simulink model "project"  (R2024b)
settings: Solver=VariableStepAuto  StartTime=0.0  StopTime=(size(Xp,2)-1)*dt  MaxStep=0.01  RelTol=1e-3
values from neighbouring files (symbols this model uses):
  Ic = I    (= 0)    [quadcopter_tmp_par.m]
  m = 4    [inertia.m]    (also in quadcopter_tmp_par.m)
  M_RB = [ m*eye(3) , zeros(3) ; zeros(3) , Ic2 ]    [inertia.m]    (also in quadcopter_tmp_par.m = [m*eye(3),zeros(3);zeros(3),Ic])
undefined symbols (not defined in the file or in its folder): alpha_P, alpha_X, alpha_Y, alpha_Z
libraries: sharedtransform x2, simulink_extras x1, sharedutil x1
settings Model: Creator=fildo7525  LastModifiedBy=vince

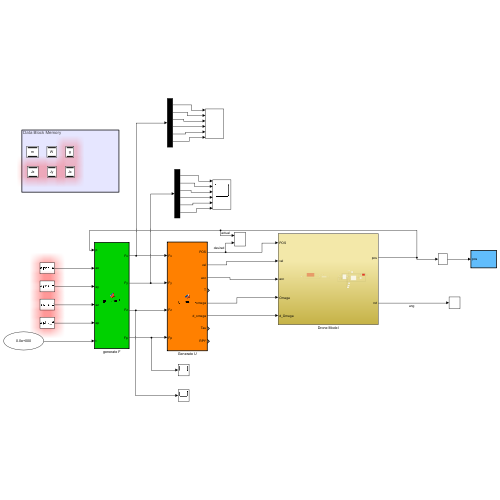
[thumbnail: Simulink's stored preview of the top-level diagram]
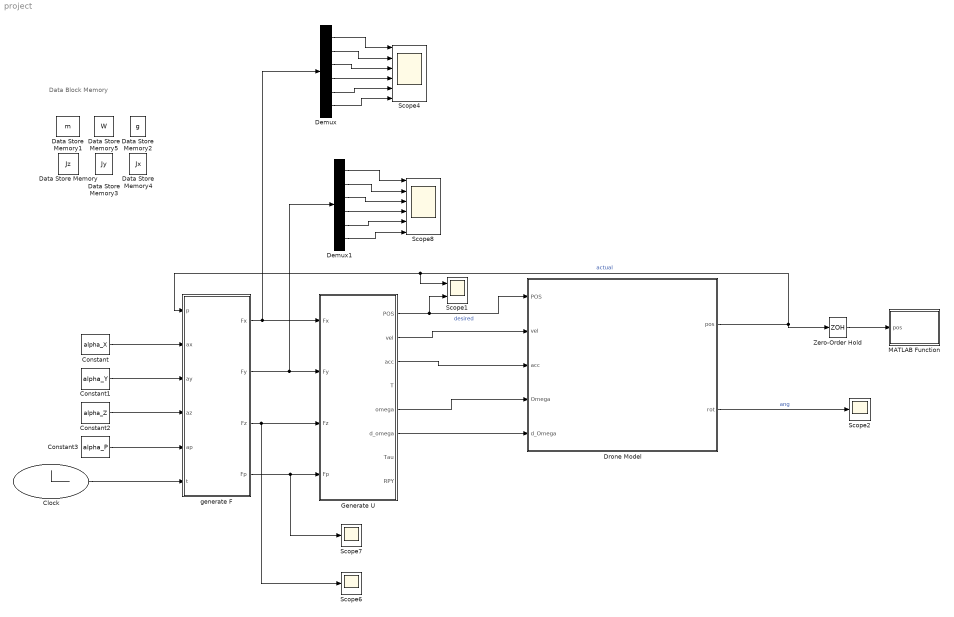
== system project ==
  note: Data Block Memory
  Clock : Clock
  Constant : Constant  Value=alpha_X
  Constant1 : Constant  Value=alpha_Y
  Constant2 : Constant  Value=alpha_Z
  Constant3 : Constant  Value=alpha_P
  Data Store Memory : DataStoreMemory  DataStoreName=Jz  WriteAfterWriteMsg=warning  InitialValue=Jz  ShowAdditionalParam=off  OutDataTypeStr=double
  Data Store Memory1 : DataStoreMemory  DataStoreName=m  WriteAfterWriteMsg=warning  InitialValue=m  ShowAdditionalParam=off  OutDataTypeStr=double
  Data Store Memory2 : DataStoreMemory  DataStoreName=g  WriteAfterWriteMsg=warning  InitialValue=g  ShowAdditionalParam=off  OutDataTypeStr=double
  Data Store Memory3 : DataStoreMemory  DataStoreName=Jy  WriteAfterWriteMsg=warning  InitialValue=Jy  ShowAdditionalParam=off  OutDataTypeStr=double
  Data Store Memory4 : DataStoreMemory  DataStoreName=Jx  WriteAfterWriteMsg=warning  InitialValue=Jx  ShowAdditionalParam=off  OutDataTypeStr=double
  Data Store Memory5 : DataStoreMemory  DataStoreName=W  WriteAfterWriteMsg=warning  InitialValue=W  ShowAdditionalParam=off  OutDataTypeStr=double
  Demux : Demux  Outputs=6
  Demux1 : Demux  Outputs=6
  Drone Model : Subsystem
  Generate U : MATLAB Function  TreatAsAtomicUnit=on
  MATLAB Function : MATLAB Function  TreatAsAtomicUnit=on
  Scope1 : Scope  NumInputPorts=2
  Scope2 : Scope
  Scope4 : Scope  NumInputPorts=6
  Scope6 : Scope
  Scope7 : Scope
  Scope8 : Scope  NumInputPorts=6
  Zero-Order Hold : ZeroOrderHold  SampleTime=0.1
  generate F : MATLAB Function  TreatAsAtomicUnit=on
  wires:
  Constant2/1 -> generate F/4(az)
  generate F/2(Fy) -> Demux1/1, Generate U/2(Fy)
  generate F/1(Fx) -> Demux/1, Generate U/1(Fx)
  Clock/1 -> generate F/6(t)
  Constant3/1 -> generate F/5(ap)
  generate F/3(Fz) -> Scope6/1, Generate U/3(Fz)
  Constant1/1 -> generate F/3(ay)
  generate F/4(Fp) -> Scope7/1, Generate U/4(Fp)
  Constant/1 -> generate F/2(ax)
  Demux/6 -> Scope4/6
  Demux/1 -> Scope4/1
  Demux/2 -> Scope4/2
  Demux/3 -> Scope4/3
  Demux/4 -> Scope4/4
  Demux/5 -> Scope4/5
  Demux1/4 -> Scope8/4
  Demux1/3 -> Scope8/3
  Demux1/1 -> Scope8/1
  Demux1/2 -> Scope8/2
  Demux1/5 -> Scope8/5
  Demux1/6 -> Scope8/6
  Drone Model/1(pos) -> Zero-Order Hold/1, Scope1/1, generate F/1(p)  "actual"
  Zero-Order Hold/1 -> MATLAB Function/1(pos)
  Drone Model/2(rot) -> Scope2/1  "ang"
  Generate U/1(POS) -> Scope1/2, Drone Model/1(POS)  "desired"
  Generate U/5(omega) -> Drone Model/4(Omega)
  Generate U/2(vel) -> Drone Model/2(vel)
  Generate U/3(acc) -> Drone Model/3(acc)
  Generate U/6(d_omega) -> Drone Model/5(d_Omega)

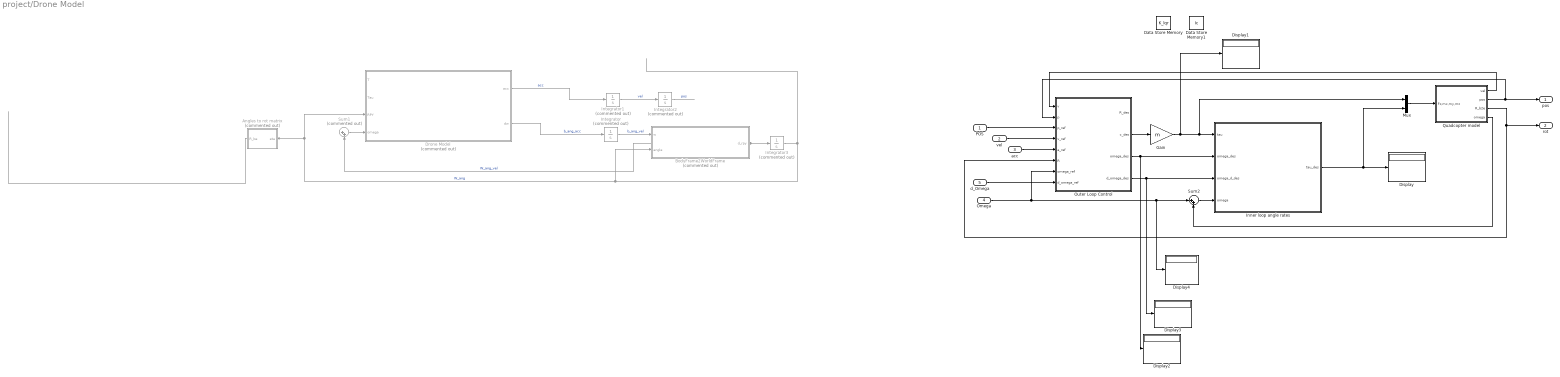
== system project/Drone Model ==
  POS : Inport
  vel : Inport  Port=2
  acc : Inport  Port=3
  Omega : Inport  Port=4
  d_Omega : Inport  Port=5
  Angles to rot matrix : MATLAB Function  Commented=on  TreatAsAtomicUnit=on
  BodyFrame2WorldFrame : MATLAB Function  Commented=on  TreatAsAtomicUnit=on
  Data Store Memory : DataStoreMemory  DataStoreName=K_lqr  WriteAfterWriteMsg=warning  InitialValue=K_lqr  VectorParams1D=off  ShowAdditionalParam=off  OutDataTypeStr=double
  Data Store Memory1 : DataStoreMemory  DataStoreName=Ic  WriteAfterWriteMsg=warning  InitialValue=Ic  VectorParams1D=off  ShowAdditionalParam=off  OutDataTypeStr=double
  Display{,1..4} (5 alike) : Display
  Drone Model : MATLAB Function  Commented=on  TreatAsAtomicUnit=on
  Gain : Gain  Gain=m
  Inner loop angle rates : MATLAB Function  TreatAsAtomicUnit=on
  Integrator{,1..3} (4 alike) : Integrator  Commented=on  InitialCondition=zeros(3,1)
  Mux : Mux  Inputs=2
  Outer Loop Control : MATLAB Function  TreatAsAtomicUnit=on
  Quadcopter model : Subsystem
  Sum1 : Sum  Commented=on  Inputs=|++
  Sum2 : Sum  Inputs=|++
  pos : Outport
  rot : Outport  Port=2
  wires:
  Integrator2/1 -> ?  "pos"
  Drone Model/1(acc) -> Integrator1/1  "acc"
  Drone Model/2(dw) -> Integrator/1  "b_ang_acc"
  Integrator1/1 -> Integrator2/1  "vel"
  BodyFrame2WorldFrame/1(d_rpy) -> Integrator3/1, Sum1/2  "W_ang_vel"
  Integrator3/1 -> Drone Model/3(RPY), Angles to rot matrix/1(eta), BodyFrame2WorldFrame/2(angle)  "W_ang"
  Integrator/1 -> BodyFrame2WorldFrame/1(w)  "b_ang_vel"
  Sum1/1 -> Drone Model/4(omega)
  Omega/1 -> Display4/1, Sum2/1, Outer Loop Control/7(omega_ref)
  POS/1 -> Outer Loop Control/3(p_ref)
  vel/1 -> Outer Loop Control/4(v_ref)
  acc/1 -> Outer Loop Control/5(a_ref)
  Angles to rot matrix/1(R_be) -> ?
  Outer Loop Control/3(omega_des) -> Inner loop angle rates/2(omega_des), Display2/1
  Outer Loop Control/4(d_omega_des) -> Display3/1, Inner loop angle rates/3(omega_d_des)
  Inner loop angle rates/1(tau_des) -> Mux/2, Display/1
  Outer Loop Control/2(c_des) -> Gain/1
  Gain/1 -> Display1/1, Mux/1, Inner loop angle rates/1(tau)
  Mux/1 -> Quadcopter model/1(Fz,mx,my,mz)
  Quadcopter model/2(pos) -> pos/1, Outer Loop Control/2(p)
  Quadcopter model/1(vel) -> Outer Loop Control/1(v)
  Quadcopter model/3(R_b2e) -> rot/1, Outer Loop Control/6(R)
  Quadcopter model/4(omega) -> Sum2/2
  Sum2/1 -> Inner loop angle rates/4(omega)
  d_Omega/1 -> Outer Loop Control/8(d_omega_ref)

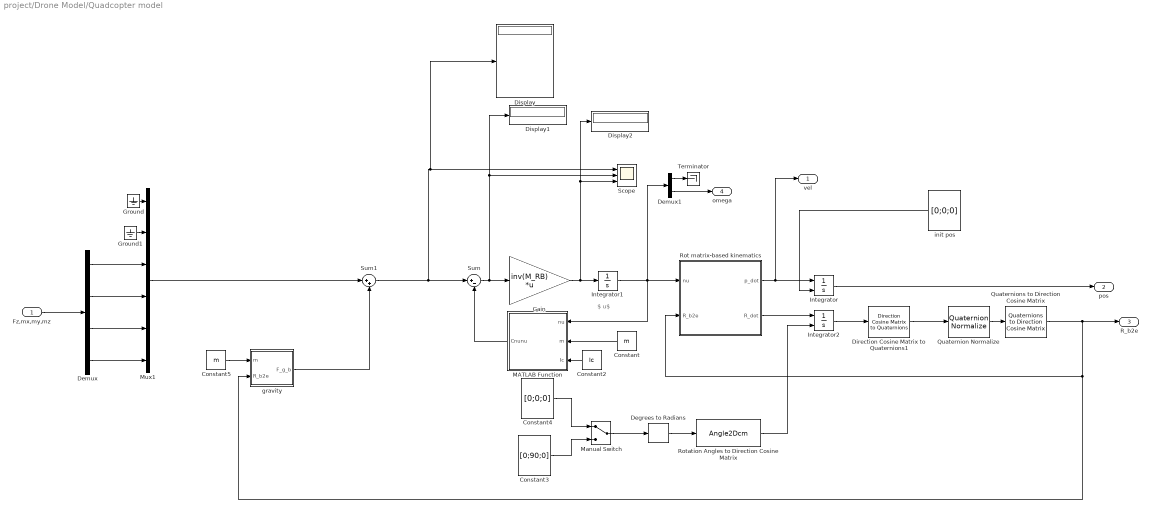
== system project/Drone Model/Quadcopter model ==
  note: $\nu$
  Fz,mx,my,mz : Inport
  Constant : Constant  Value=m
  Constant2 : Constant  Value=Ic  VectorParams1D=off
  Constant3 : Constant  Value=[0;90;0]  VectorParams1D=off
  Constant4 : Constant  Value=[0;0;0]  VectorParams1D=off
  Constant5 : Constant  Value=m
  Degrees to Radians : simulink_extras/Transformations/Degrees to Radians
  Demux : Demux
  Demux1 : Demux  Outputs=2
  Direction Cosine Matrix to Quaternions1 : sharedtransform/Direction Cosine Matrix  to Quaternions  aMode=0  action=None  tolerance=eps(2)
  Display : Display
      settings: Decimation=3
  Display1 : Display
      settings: Decimation=3
  Display2 : Display
      settings: Decimation=3
  Gain : Gain  Gain=inv(M_RB)  Multiplication=Matrix(K*u) (u vector)
  Ground : Ground
  Ground1 : Ground
  Integrator : Integrator  InitialConditionSource=external  InitialCondition=[0;0;-10]
  Integrator1 : Integrator  InitialCondition=[0;0;0;0;0;0]
  Integrator2 : Integrator  InitialConditionSource=external  InitialCondition=[0;0;-10;0;pi/2;0]
  MATLAB Function : MATLAB Function  TreatAsAtomicUnit=on
  Manual Switch : ManualSwitch
  Mux1 : Mux  Inputs=6
  Quaternion Normalize : sharedutil/Quaternion Normalize  aMode=aMode
  Quaternions to Direction Cosine Matrix : sharedtransform/Quaternions to  Direction Cosine Matrix  aMode=aMode
  Rot matrix-based kinematics : Subsystem
  Rotation Angles to Direction Cosine Matrix : Angle2Dcm
      settings: AttributesFormatString=Rotation Order: %<rotationOrder>
  Scope : Scope  NumInputPorts=3
  Sum : Sum  Inputs=|+-
  Sum1 : Sum  Inputs=|++
  Terminator : Terminator
  gravity : MATLAB Function  TreatAsAtomicUnit=on
  init pos : Constant  Value=[0;0;0]  VectorParams1D=off
  vel : Outport
  pos : Outport  Port=2
  R_b2e : Outport  Port=3
  omega : Outport  Port=4
  wires:
  Constant/1 -> MATLAB Function/2(m)
  Degrees to Radians/1 -> Rotation Angles to Direction Cosine Matrix/1
  Constant2/1 -> MATLAB Function/3(Ic)
  init pos/1 -> Integrator/2
  Constant4/1 -> Manual Switch/1
  MATLAB Function/1(Cnunu) -> Sum/2
  Gain/1 -> Display2/1, Scope/3, Integrator1/1
  Constant3/1 -> Manual Switch/2
  Rotation Angles to Direction Cosine Matrix/1 -> Integrator2/2
  Sum/1 -> Scope/2, Display1/1, Gain/1
  Manual Switch/1 -> Degrees to Radians/1
  Rot matrix-based kinematics/1(p_dot) -> Integrator/1, vel/1
  Rot matrix-based kinematics/2(R_dot) -> Integrator2/1
  Integrator/1 -> pos/1
  Demux/4 -> Mux1/6
  Demux/3 -> Mux1/5
  Demux/2 -> Mux1/4
  Fz,mx,my,mz/1 -> Demux/1
  Ground/1 -> Mux1/1
  Ground1/1 -> Mux1/2
  Quaternion Normalize/1 -> Quaternions to Direction Cosine Matrix/1
  Constant5/1 -> gravity/1(m)
  gravity/1(F_g_b) -> Sum1/2
  Sum1/1 -> Display/1, Scope/1, Sum/1
  Demux/1 -> Mux1/3
  Integrator1/1 -> Demux1/1, MATLAB Function/1(nu), Rot matrix-based kinematics/1(nu)
  Direction Cosine Matrix to Quaternions1/1 -> Quaternion Normalize/1
  Quaternions to Direction Cosine Matrix/1 -> gravity/2(R_b2e), Rot matrix-based kinematics/2(R_b2e), R_b2e/1
  Integrator2/1 -> Direction Cosine Matrix to Quaternions1/1
  Mux1/1 -> Sum1/1
  Demux1/1 -> Terminator/1
  Demux1/2 -> omega/1

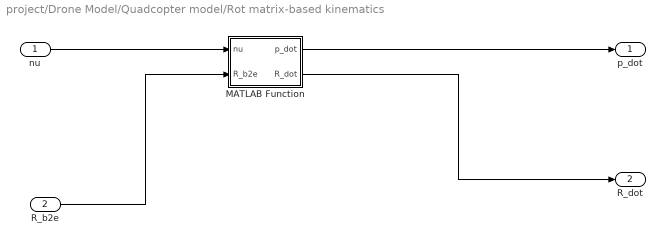
== system project/Drone Model/Quadcopter model/Rot matrix-based kinematics ==
  nu : Inport
  R_b2e : Inport  Port=2
  MATLAB Function : MATLAB Function  TreatAsAtomicUnit=on
  p_dot : Outport
  R_dot : Outport  Port=2
  wires:
  MATLAB Function/2(R_dot) -> R_dot/1
  nu/1 -> MATLAB Function/1(nu)
  R_b2e/1 -> MATLAB Function/2(R_b2e)
  MATLAB Function/1(p_dot) -> p_dot/1

== matlab function project/Drone Model/Angles to rot matrix ==
  data: R_be output; eta input
function R_be = fcn(eta)

% Euler angle extraction
phi = eta(4);
theta = eta(5);
psi = eta(6);

R_xphi = [ 1 0 0 ; 0 cos(phi) -sin(phi) ; 0 sin(phi) cos(phi) ];
R_ytheta = [ cos(theta) 0 sin(theta) ; 0 1 0 ; -sin(theta) 0 cos(theta) ];
R_zpsi = [ cos(psi) -sin(psi) 0 ; sin(psi) cos(psi) 0 ; 0 0 1 ];

% rotation matrix
R_be = R_zpsi * R_ytheta * R_xphi;

== matlab function project/Drone Model/BodyFrame2WorldFrame ==
  data: d_rpy output; w input; angle input
function d_rpy = convertBodyFrame2WorldFrame(w, angle)
	Fi = angle(1);
	Theta = angle(2);
	Psi = angle(3);

	R = [1, 0		, -sin(Theta);
		 0, cos(Fi) , cos(Theta)*sin(Fi);
		 0, -sin(Fi), cos(Theta)*cos(Fi)];

	d_rpy = R \ w;

== matlab function project/Drone Model/Quadcopter model/MATLAB Function ==
  data: nu input; Cnunu output; m input; Ic input
function Cnunu = fcn(nu,m,Ic)

v = nu(1:3);  % linear velocities (expressed in the body frame)
omega = nu(4:6); % angular velocities (expressed in the body frame)

% Coriolis term
Cnunu = [ cross(omega,m*v) ; -cross(Ic*omega,omega) ];

== matlab function project/Drone Model/Quadcopter model/gravity ==
  data: m input; R_b2e input; F_g_b output
function F_g_b = fcn(m,R_b2e)
F_g=[0;0;-m*9.81];
F_g_b=[R_b2e'*F_g;0;0;0];

== matlab function project/Drone Model/Quadcopter model/Rot matrix-based kinematics/MATLAB Function ==
  data: nu input; p_dot output; R_b2e input; R_dot output
function [p_dot,R_dot] = fcn(nu,R_b2e)
v_b=nu(1:3);
w_b=nu(4:6);
p_dot=R_b2e*v_b;
omega_cross=[0,-w_b(3),w_b(2);
             w_b(3),0,-w_b(1);
             -w_b(2),w_b(1),0];
R_dot=R_b2e*omega_cross;

== matlab function project/Drone Model/Inner loop angle rates ==
  settings: updateMethod=DISCRETE
  data: tau input; omega_des input; omega_d_des input; omega input; tau_des output; Ic data_store_memory; K_lqr data_store_memory
function tau_des = inner(tau, omega_des, omega_d_des, omega)
	global K_lqr;
	global Ic;

	tau_ref = cross(omega_des, Ic*omega_des) + Ic*omega_d_des;
	
	tau_des = K_lqr * [omega_des-omega; tau_ref-tau] + cross(omega, Ic*omega) + Ic * omega_d_des;

== matlab function project/generate F ==
  settings: updateMethod=DISCRETE
  data: p input; ax input; Fx output; ay input; az input; ap input; t input; Fy output; Fz output; Fp output; W data_store_memory
function [Fx, Fy, Fz, Fp] = generateF(p, ax, ay, az, ap, t)
    global W;
    
    persistent acceptance;
	persistent idx;

    if isempty(idx)
		idx = 1;
        % acceptance = 0.2;
		acceptance = 0.5;
    end

	b0 = [ 1 ; t ; t^2	; t^3	; t^4	 ; t^5];
	b1 = [ 0 ; 1 ; 2*t	; 3*t^2 ; 4*t^3	 ; 5*t^4];
    b2 = [ 0 ; 0 ; 2	; 6*t	; 12*t^2 ; 20*t^3];
	b3 = [ 0 ; 0 ; 0	; 6		; 24*t	 ; 60*t^2];
	b4 = [ 0 ; 0 ; 0	; 0		; 24	 ; 120*t];
	b5 = [ 0 ; 0 ; 0	; 0		; 0		 ; 120];
    
    Fx = [ax(idx, :)*b0; ax(idx, :)*b1; ax(idx, :)*b2; ax(idx, :)*b3; ax(idx, :)*b4; ax(idx, :)*b5];
    Fy = [ay(idx, :)*b0; ay(idx, :)*b1; ay(idx, :)*b2; ay(idx, :)*b3; ay(idx, :)*b4; ay(idx, :)*b5];
    Fz = [az(idx, :)*b0; az(idx, :)*b1; az(idx, :)*b2; az(idx, :)*b3; az(idx, :)*b4; az(idx, :)*b5];
    Fp = [ap(idx, :)*b0; ap(idx, :)*b1; ap(idx, :)*b2; ap(idx, :)*b3; ap(idx, :)*b4; ap(idx, :)*b5];

    %v = K*(pd - p) Fi,
	dif = norm(W(idx+1, 1:3) - p');
    if dif <= acceptance
		if idx + 1 < size(W, 1)
			idx = idx + 1;
		end
	end

end

== matlab function project/Generate U ==
  data: POS output; vel output; acc output; Fx input; T output; omega output; d_omega output; Tau output; RPY output; Fy input; Fz input; Fp input; Jz data_store_memory; g data_store_memory; m data_store_memory; Jx data_store_memory; Jy data_store_memory
function [POS, vel, acc, T, omega, d_omega, Tau, RPY] = generateU(Fx, Fy, Fz, Fp)
    global Jz;
    global Jy;
    global Jx;
    global m;
    global g;
    
    f1c4f2s4 = Fx(3) * cos(Fp(1)) + Fy(3) * sin(Fp(1));
    
    T = m * sqrt( Fx(3)^2 + Fy(3)^2 + (Fz(3) + g)^2 );
	POS = [Fx(1); Fy(1); Fz(1)];
	vel = [Fx(1); Fy(1); Fz(1)];
	acc = [Fx(1); Fy(1); Fz(1)];
	
	Psi = Fp(1);
	tmp = Fx(3)*cos(Psi) + Fy(3)*sin(Psi);
	Theta = atan2( tmp, Fz(3) + g );
	Fi = atan2( Fx(3)*sin(Psi) - Fy(3)*cos(Psi), sqrt( (Fz(3)+g)^2 + tmp^2) );
	
	RPY = [ Fi; Theta; Psi];


	wx = ((sin(Fp(1))*Fx(4) - cos(Fp(1))*Fy(4) + cos(Fp(1))*Fx(3)*Fp(2) + sin(Fp(1))*Fy(3)*Fp(2))/((Fz(3) + g)^2 + (cos(Fp(1))*Fx(3) + sin(Fp(1))*Fy(3))^2)^(1/2) + ((2*(Fz(3) + g)*Fz(4) + 2*(cos(Fp(1))*Fx(3) + sin(Fp(1))*Fy(3))*(sin(Fp(1))*Fy(4) + cos(Fp(1))*Fx(4) + cos(Fp(1))*Fy(3)*Fp(2) - sin(Fp(1))*Fx(3)*Fp(2)))*(cos(Fp(1))*Fy(3) - sin(Fp(1))*Fx(3)))/(2*((Fz(3) + g)^2 + (cos(Fp(1))*Fx(3) + sin(Fp(1))*Fy(3))^2)^(3/2)))/((cos(Fp(1))*Fy(3) - sin(Fp(1))*Fx(3))^2/((Fz(3) + g)^2 + (cos(Fp(1))*Fx(3) + sin(Fp(1))*Fy(3))^2) + 1) - ((cos(Fp(1))*Fx(3) + sin(Fp(1))*Fy(3))*Fp(2))/(((cos(Fp(1))*Fx(3) + sin(Fp(1))*Fy(3))^2/(Fz(3) + g)^2 + 1)^(1/2)*(Fz(3) + g));
	wy = ((sin(Fp(1))*Fy(4) + cos(Fp(1))*Fx(4) + cos(Fp(1))*Fy(3)*Fp(2) - sin(Fp(1))*Fx(3)*Fp(2))/(Fz(3) + g) - ((cos(Fp(1))*Fx(3) + sin(Fp(1))*Fy(3))*Fz(4))/(Fz(3) + g)^2)/(((cos(Fp(1))*Fx(3) + sin(Fp(1))*Fy(3))^2/(Fz(3) + g)^2 + 1)*((cos(Fp(1))*Fy(3) - sin(Fp(1))*Fx(3))^2/((Fz(3) + g)^2 + (cos(Fp(1))*Fx(3) + sin(Fp(1))*Fy(3))^2) + 1)^(1/2)) - ((cos(Fp(1))*Fy(3) - sin(Fp(1))*Fx(3))*Fp(2))/(((cos(Fp(1))*Fx(3) + sin(Fp(1))*Fy(3))^2/(Fz(3) + g)^2 + 1)^(1/2)*((cos(Fp(1))*Fy(3) - sin(Fp(1))*Fx(3))^2/((Fz(3) + g)^2 + (cos(Fp(1))*Fx(3) + sin(Fp(1))*Fy(3))^2) + 1)^(1/2)*((Fz(3) + g)^2 + (cos(Fp(1))*Fx(3) + sin(Fp(1))*Fy(3))^2)^(1/2));
	wz = Fp(2)/(((cos(Fp(1))*Fx(3) + sin(Fp(1))*Fy(3))^2/(Fz(3) + g)^2 + 1)^(1/2)*((cos(Fp(1))*Fy(3) - sin(Fp(1))*Fx(3))^2/((Fz(3) + g)^2 + (cos(Fp(1))*Fx(3) + sin(Fp(1))*Fy(3))^2) + 1)^(1/2)) + (((sin(Fp(1))*Fy(4) + cos(Fp(1))*Fx(4) + cos(Fp(1))*Fy(3)*Fp(2) - sin(Fp(1))*Fx(3)*Fp(2))/(Fz(3) + g) - ((cos(Fp(1))*Fx(3) + sin(Fp(1))*Fy(3))*Fz(4))/(Fz(3) + g)^2)*(cos(Fp(1))*Fy(3) - sin(Fp(1))*Fx(3)))/(((cos(Fp(1))*Fx(3) + sin(Fp(1))*Fy(3))^2/(Fz(3) + g)^2 + 1)*((cos(Fp(1))*Fy(3) - sin(Fp(1))*Fx(3))^2/((Fz(3) + g)^2 + (cos(Fp(1))*Fx(3) + sin(Fp(1))*Fy(3))^2) + 1)^(1/2)*((Fz(3) + g)^2 + (cos(Fp(1))*Fx(3) + sin(Fp(1))*Fy(3))^2)^(1/2));

	omega = [wx; wy; wz];

	dwx = ((sin(Fp(1))*Fx(5) - cos(Fp(1))*Fy(5) + cos(Fp(1))*Fp(2)^2*Fy(3) - sin(Fp(1))*Fp(2)^2*Fx(3) + 2*cos(Fp(1))*Fp(2)*Fx(4) + cos(Fp(1))*Fp(3)*Fx(3) + 2*sin(Fp(1))*Fp(2)*Fy(4) + sin(Fp(1))*Fp(3)*Fy(3))/((Fz(3) + g)^2 + (cos(Fp(1))*Fx(3) + sin(Fp(1))*Fy(3))^2)^(1/2) + ((cos(Fp(1))*Fy(3) - sin(Fp(1))*Fx(3))*(2*(cos(Fp(1))*Fx(3) + sin(Fp(1))*Fy(3))*(cos(Fp(1))*Fx(5) + sin(Fp(1))*Fy(5) - cos(Fp(1))*Fp(2)^2*Fx(3) - sin(Fp(1))*Fp(2)^2*Fy(3) + 2*cos(Fp(1))*Fp(2)*Fy(4) + cos(Fp(1))*Fp(3)*Fy(3) - 2*sin(Fp(1))*Fp(2)*Fx(4) - sin(Fp(1))*Fp(3)*Fx(3)) + 2*(Fz(3) + g)*Fz(5) + 2*Fz(4)^2 + 2*(sin(Fp(1))*Fy(4) + cos(Fp(1))*Fx(4) + cos(Fp(1))*Fy(3)*Fp(2) - sin(Fp(1))*Fx(3)*Fp(2))^2))/(2*((Fz(3) + g)^2 + (cos(Fp(1))*Fx(3) + sin(Fp(1))*Fy(3))^2)^(3/2)) - ((2*(Fz(3) + g)*Fz(4) + 2*(cos(Fp(1))*Fx(3) + sin(Fp(1))*Fy(3))*(sin(Fp(1))*Fy(4) + cos(Fp(1))*Fx(4) + cos(Fp(1))*Fy(3)*Fp(2) - sin(Fp(1))*Fx(3)*Fp(2)))*(sin(Fp(1))*Fx(4) - cos(Fp(1))*Fy(4) + cos(Fp(1))*Fx(3)*Fp(2) + sin(Fp(1))*Fy(3)*Fp(2)))/((Fz(3) + g)^2 + (cos(Fp(1))*Fx(3) + sin(Fp(1))*Fy(3))^2)^(3/2) - (3*(2*(Fz(3) + g)*Fz(4) + 2*(cos(Fp(1))*Fx(3) + sin(Fp(1))*Fy(3))*(sin(Fp(1))*Fy(4) + cos(Fp(1))*Fx(4) + cos(Fp(1))*Fy(3)*Fp(2) - sin(Fp(1))*Fx(3)*Fp(2)))^2*(cos(Fp(1))*Fy(3) - sin(Fp(1))*Fx(3)))/(4*((Fz(3) + g)^2 + (cos(Fp(1))*Fx(3) + sin(Fp(1))*Fy(3))^2)^(5/2)))/((cos(Fp(1))*Fy(3) - sin(Fp(1))*Fx(3))^2/((Fz(3) + g)^2 + (cos(Fp(1))*Fx(3) + sin(Fp(1))*Fy(3))^2) + 1) + (((sin(Fp(1))*Fx(4) - cos(Fp(1))*Fy(4) + cos(Fp(1))*Fx(3)*Fp(2) + sin(Fp(1))*Fy(3)*Fp(2))/((Fz(3) + g)^2 + (cos(Fp(1))*Fx(3) + sin(Fp(1))*Fy(3))^2)^(1/2) + ((2*(Fz(3) + g)*Fz(4) + 2*(cos(Fp(1))*Fx(3) + sin(Fp(1))*Fy(3))*(sin(Fp(1))*Fy(4) + cos(Fp(1))*Fx(4) + cos(Fp(1))*Fy(3)*Fp(2) - sin(Fp(1))*Fx(3)*Fp(2)))*(cos(Fp(1))*Fy(3) - sin(Fp(1))*Fx(3)))/(2*((Fz(3) + g)^2 + (cos(Fp(1))*Fx(3) + sin(Fp(1))*Fy(3))^2)^(3/2)))*(((2*(Fz(3) + g)*Fz(4) + 2*(cos(Fp(1))*Fx(3) + sin(Fp(1))*Fy(3))*(sin(Fp(1))*Fy(4) + cos(Fp(1))*Fx(4) + cos(Fp(1))*Fy(3)*Fp(2) - sin(Fp(1))*Fx(3)*Fp(2)))*(cos(Fp(1))*Fy(3) - sin(Fp(1))*Fx(3))^2)/((Fz(3) + g)^2 + (cos(Fp(1))*Fx(3) + sin(Fp(1))*Fy(3))^2)^2 + (2*(cos(Fp(1))*Fy(3) - sin(Fp(1))*Fx(3))*(sin(Fp(1))*Fx(4) - cos(Fp(1))*Fy(4) + cos(Fp(1))*Fx(3)*Fp(2) + sin(Fp(1))*Fy(3)*Fp(2)))/((Fz(3) + g)^2 + (cos(Fp(1))*Fx(3) + sin(Fp(1))*Fy(3))^2)))/((cos(Fp(1))*Fy(3) - sin(Fp(1))*Fx(3))^2/((Fz(3) + g)^2 + (cos(Fp(1))*Fx(3) + sin(Fp(1))*Fy(3))^2) + 1)^2 - (Fp(2)*(sin(Fp(1))*Fy(4) + cos(Fp(1))*Fx(4) + cos(Fp(1))*Fy(3)*Fp(2) - sin(Fp(1))*Fx(3)*Fp(2)))/(((cos(Fp(1))*Fx(3) + sin(Fp(1))*Fy(3))^2/(Fz(3) + g)^2 + 1)^(1/2)*(Fz(3) + g)) - ((cos(Fp(1))*Fx(3) + sin(Fp(1))*Fy(3))*Fp(3))/(((cos(Fp(1))*Fx(3) + sin(Fp(1))*Fy(3))^2/(Fz(3) + g)^2 + 1)^(1/2)*(Fz(3) + g)) + ((cos(Fp(1))*Fx(3) + sin(Fp(1))*Fy(3))*Fp(2)*Fz(4))/(((cos(Fp(1))*Fx(3) + sin(Fp(1))*Fy(3))^2/(Fz(3) + g)^2 + 1)^(1/2)*(Fz(3) + g)^2) + (((2*(cos(Fp(1))*Fx(3) + sin(Fp(1))*Fy(3))*(sin(Fp(1))*Fy(4) + cos(Fp(1))*Fx(4) + cos(Fp(1))*Fy(3)*Fp(2) - sin(Fp(1))*Fx(3)*Fp(2)))/(Fz(3) + g)^2 - (2*(cos(Fp(1))*Fx(3) + sin(Fp(1))*Fy(3))^2*Fz(4))/(Fz(3) + g)^3)*(cos(Fp(1))*Fx(3) + sin(Fp(1))*Fy(3))*Fp(2))/(2*((cos(Fp(1))*Fx(3) + sin(Fp(1))*Fy(3))^2/(Fz(3) + g)^2 + 1)^(3/2)*(Fz(3) + g));
	dwy = ((cos(Fp(1))*Fx(5) + sin(Fp(1))*Fy(5) - cos(Fp(1))*Fp(2)^2*Fx(3) - sin(Fp(1))*Fp(2)^2*Fy(3) + 2*cos(Fp(1))*Fp(2)*Fy(4) + cos(Fp(1))*Fp(3)*Fy(3) - 2*sin(Fp(1))*Fp(2)*Fx(4) - sin(Fp(1))*Fp(3)*Fx(3))/(Fz(3) + g) - (2*Fz(4)*(sin(Fp(1))*Fy(4) + cos(Fp(1))*Fx(4) + cos(Fp(1))*Fy(3)*Fp(2) - sin(Fp(1))*Fx(3)*Fp(2)))/(Fz(3) + g)^2 + (2*(cos(Fp(1))*Fx(3) + sin(Fp(1))*Fy(3))*Fz(4)^2)/(Fz(3) + g)^3 - ((cos(Fp(1))*Fx(3) + sin(Fp(1))*Fy(3))*Fz(5))/(Fz(3) + g)^2)/(((cos(Fp(1))*Fx(3) + sin(Fp(1))*Fy(3))^2/(Fz(3) + g)^2 + 1)*((cos(Fp(1))*Fy(3) - sin(Fp(1))*Fx(3))^2/((Fz(3) + g)^2 + (cos(Fp(1))*Fx(3) + sin(Fp(1))*Fy(3))^2) + 1)^(1/2)) + (((sin(Fp(1))*Fy(4) + cos(Fp(1))*Fx(4) + cos(Fp(1))*Fy(3)*Fp(2) - sin(Fp(1))*Fx(3)*Fp(2))/(Fz(3) + g) - ((cos(Fp(1))*Fx(3) + sin(Fp(1))*Fy(3))*Fz(4))/(Fz(3) + g)^2)*(((2*(Fz(3) + g)*Fz(4) + 2*(cos(Fp(1))*Fx(3) + sin(Fp(1))*Fy(3))*(sin(Fp(1))*Fy(4) + cos(Fp(1))*Fx(4) + cos(Fp(1))*Fy(3)*Fp(2) - sin(Fp(1))*Fx(3)*Fp(2)))*(cos(Fp(1))*Fy(3) - sin(Fp(1))*Fx(3))^2)/((Fz(3) + g)^2 + (cos(Fp(1))*Fx(3) + sin(Fp(1))*Fy(3))^2)^2 + (2*(cos(Fp(1))*Fy(3) - sin(Fp(1))*Fx(3))*(sin(Fp(1))*Fx(4) - cos(Fp(1))*Fy(4) + cos(Fp(1))*Fx(3)*Fp(2) + sin(Fp(1))*Fy(3)*Fp(2)))/((Fz(3) + g)^2 + (cos(Fp(1))*Fx(3) + sin(Fp(1))*Fy(3))^2)))/(2*((cos(Fp(1))*Fx(3) + sin(Fp(1))*Fy(3))^2/(Fz(3) + g)^2 + 1)*((cos(Fp(1))*Fy(3) - sin(Fp(1))*Fx(3))^2/((Fz(3) + g)^2 + (cos(Fp(1))*Fx(3) + sin(Fp(1))*Fy(3))^2) + 1)^(3/2)) - (((2*(cos(Fp(1))*Fx(3) + sin(Fp(1))*Fy(3))*(sin(Fp(1))*Fy(4) + cos(Fp(1))*Fx(4) + cos(Fp(1))*Fy(3)*Fp(2) - sin(Fp(1))*Fx(3)*Fp(2)))/(Fz(3) + g)^2 - (2*(cos(Fp(1))*Fx(3) + sin(Fp(1))*Fy(3))^2*Fz(4))/(Fz(3) + g)^3)*((sin(Fp(1))*Fy(4) + cos(Fp(1))*Fx(4) + cos(Fp(1))*Fy(3)*Fp(2) - sin(Fp(1))*Fx(3)*Fp(2))/(Fz(3) + g) - ((cos(Fp(1))*Fx(3) + sin(Fp(1))*Fy(3))*Fz(4))/(Fz(3) + g)^2))/(((cos(Fp(1))*Fx(3) + sin(Fp(1))*Fy(3))^2/(Fz(3) + g)^2 + 1)^2*((cos(Fp(1))*Fy(3) - sin(Fp(1))*Fx(3))^2/((Fz(3) + g)^2 + (cos(Fp(1))*Fx(3) + sin(Fp(1))*Fy(3))^2) + 1)^(1/2)) - ((cos(Fp(1))*Fy(3) - sin(Fp(1))*Fx(3))*Fp(3))/(((cos(Fp(1))*Fx(3) + sin(Fp(1))*Fy(3))^2/(Fz(3) + g)^2 + 1)^(1/2)*((cos(Fp(1))*Fy(3) - sin(Fp(1))*Fx(3))^2/((Fz(3) + g)^2 + (cos(Fp(1))*Fx(3) + sin(Fp(1))*Fy(3))^2) + 1)^(1/2)*((Fz(3) + g)^2 + (cos(Fp(1))*Fx(3) + sin(Fp(1))*Fy(3))^2)^(1/2)) + (Fp(2)*(sin(Fp(1))*Fx(4) - cos(Fp(1))*Fy(4) + cos(Fp(1))*Fx(3)*Fp(2) + sin(Fp(1))*Fy(3)*Fp(2)))/(((cos(Fp(1))*Fx(3) + sin(Fp(1))*Fy(3))^2/(Fz(3) + g)^2 + 1)^(1/2)*((cos(Fp(1))*Fy(3) - sin(Fp(1))*Fx(3))^2/((Fz(3) + g)^2 + (cos(Fp(1))*Fx(3) + sin(Fp(1))*Fy(3))^2) + 1)^(1/2)*((Fz(3) + g)^2 + (cos(Fp(1))*Fx(3) + sin(Fp(1))*Fy(3))^2)^(1/2)) - ((cos(Fp(1))*Fy(3) - sin(Fp(1))*Fx(3))*Fp(2)*(((2*(Fz(3) + g)*Fz(4) + 2*(cos(Fp(1))*Fx(3) + sin(Fp(1))*Fy(3))*(sin(Fp(1))*Fy(4) + cos(Fp(1))*Fx(4) + cos(Fp(1))*Fy(3)*Fp(2) - sin(Fp(1))*Fx(3)*Fp(2)))*(cos(Fp(1))*Fy(3) - sin(Fp(1))*Fx(3))^2)/((Fz(3) + g)^2 + (cos(Fp(1))*Fx(3) + sin(Fp(1))*Fy(3))^2)^2 + (2*(cos(Fp(1))*Fy(3) - sin(Fp(1))*Fx(3))*(sin(Fp(1))*Fx(4) - cos(Fp(1))*Fy(4) + cos(Fp(1))*Fx(3)*Fp(2) + sin(Fp(1))*Fy(3)*Fp(2)))/((Fz(3) + g)^2 + (cos(Fp(1))*Fx(3) + sin(Fp(1))*Fy(3))^2)))/(2*((cos(Fp(1))*Fx(3) + sin(Fp(1))*Fy(3))^2/(Fz(3) + g)^2 + 1)^(1/2)*((cos(Fp(1))*Fy(3) - sin(Fp(1))*Fx(3))^2/((Fz(3) + g)^2 + (cos(Fp(1))*Fx(3) + sin(Fp(1))*Fy(3))^2) + 1)^(3/2)*((Fz(3) + g)^2 + (cos(Fp(1))*Fx(3) + sin(Fp(1))*Fy(3))^2)^(1/2)) + (((2*(cos(Fp(1))*Fx(3) + sin(Fp(1))*Fy(3))*(sin(Fp(1))*Fy(4) + cos(Fp(1))*Fx(4) + cos(Fp(1))*Fy(3)*Fp(2) - sin(Fp(1))*Fx(3)*Fp(2)))/(Fz(3) + g)^2 - (2*(cos(Fp(1))*Fx(3) + sin(Fp(1))*Fy(3))^2*Fz(4))/(Fz(3) + g)^3)*(cos(Fp(1))*Fy(3) - sin(Fp(1))*Fx(3))*Fp(2))/(2*((cos(Fp(1))*Fx(3) + sin(Fp(1))*Fy(3))^2/(Fz(3) + g)^2 + 1)^(3/2)*((cos(Fp(1))*Fy(3) - sin(Fp(1))*Fx(3))^2/((Fz(3) + g)^2 + (cos(Fp(1))*Fx(3) + sin(Fp(1))*Fy(3))^2) + 1)^(1/2)*((Fz(3) + g)^2 + (cos(Fp(1))*Fx(3) + sin(Fp(1))*Fy(3))^2)^(1/2)) + ((2*(Fz(3) + g)*Fz(4) + 2*(cos(Fp(1))*Fx(3) + sin(Fp(1))*Fy(3))*(sin(Fp(1))*Fy(4) + cos(Fp(1))*Fx(4) + cos(Fp(1))*Fy(3)*Fp(2) - sin(Fp(1))*Fx(3)*Fp(2)))*(cos(Fp(1))*Fy(3) - sin(Fp(1))*Fx(3))*Fp(2))/(2*((cos(Fp(1))*Fx(3) + sin(Fp(1))*Fy(3))^2/(Fz(3) + g)^2 + 1)^(1/2)*((cos(Fp(1))*Fy(3) - sin(Fp(1))*Fx(3))^2/((Fz(3) + g)^2 + (cos(Fp(1))*Fx(3) + sin(Fp(1))*Fy(3))^2) + 1)^(1/2)*((Fz(3) + g)^2 + (cos(Fp(1))*Fx(3) + sin(Fp(1))*Fy(3))^2)^(3/2));
	dwz = Fp(3)/(((cos(Fp(1))*Fx(3) + sin(Fp(1))*Fy(3))^2/(Fz(3) + g)^2 + 1)^(1/2)*((cos(Fp(1))*Fy(3) - sin(Fp(1))*Fx(3))^2/((Fz(3) + g)^2 + (cos(Fp(1))*Fx(3) + sin(Fp(1))*Fy(3))^2) + 1)^(1/2)) - (((2*(cos(Fp(1))*Fx(3) + sin(Fp(1))*Fy(3))*(sin(Fp(1))*Fy(4) + cos(Fp(1))*Fx(4) + cos(Fp(1))*Fy(3)*Fp(2) - sin(Fp(1))*Fx(3)*Fp(2)))/(Fz(3) + g)^2 - (2*(cos(Fp(1))*Fx(3) + sin(Fp(1))*Fy(3))^2*Fz(4))/(Fz(3) + g)^3)*Fp(2))/(2*((cos(Fp(1))*Fx(3) + sin(Fp(1))*Fy(3))^2/(Fz(3) + g)^2 + 1)^(3/2)*((cos(Fp(1))*Fy(3) - sin(Fp(1))*Fx(3))^2/((Fz(3) + g)^2 + (cos(Fp(1))*Fx(3) + sin(Fp(1))*Fy(3))^2) + 1)^(1/2)) + (Fp(2)*(((2*(Fz(3) + g)*Fz(4) + 2*(cos(Fp(1))*Fx(3) + sin(Fp(1))*Fy(3))*(sin(Fp(1))*Fy(4) + cos(Fp(1))*Fx(4) + cos(Fp(1))*Fy(3)*Fp(2) - sin(Fp(1))*Fx(3)*Fp(2)))*(cos(Fp(1))*Fy(3) - sin(Fp(1))*Fx(3))^2)/((Fz(3) + g)^2 + (cos(Fp(1))*Fx(3) + sin(Fp(1))*Fy(3))^2)^2 + (2*(cos(Fp(1))*Fy(3) - sin(Fp(1))*Fx(3))*(sin(Fp(1))*Fx(4) - cos(Fp(1))*Fy(4) + cos(Fp(1))*Fx(3)*Fp(2) + sin(Fp(1))*Fy(3)*Fp(2)))/((Fz(3) + g)^2 + (cos(Fp(1))*Fx(3) + sin(Fp(1))*Fy(3))^2)))/(2*((cos(Fp(1))*Fx(3) + sin(Fp(1))*Fy(3))^2/(Fz(3) + g)^2 + 1)^(1/2)*((cos(Fp(1))*Fy(3) - sin(Fp(1))*Fx(3))^2/((Fz(3) + g)^2 + (cos(Fp(1))*Fx(3) + sin(Fp(1))*Fy(3))^2) + 1)^(3/2)) + ((cos(Fp(1))*Fy(3) - sin(Fp(1))*Fx(3))*((cos(Fp(1))*Fx(5) + sin(Fp(1))*Fy(5) - cos(Fp(1))*Fp(2)^2*Fx(3) - sin(Fp(1))*Fp(2)^2*Fy(3) + 2*cos(Fp(1))*Fp(2)*Fy(4) + cos(Fp(1))*Fp(3)*Fy(3) - 2*sin(Fp(1))*Fp(2)*Fx(4) - sin(Fp(1))*Fp(3)*Fx(3))/(Fz(3) + g) - (2*Fz(4)*(sin(Fp(1))*Fy(4) + cos(Fp(1))*Fx(4) + cos(Fp(1))*Fy(3)*Fp(2) - sin(Fp(1))*Fx(3)*Fp(2)))/(Fz(3) + g)^2 + (2*(cos(Fp(1))*Fx(3) + sin(Fp(1))*Fy(3))*Fz(4)^2)/(Fz(3) + g)^3 - ((cos(Fp(1))*Fx(3) + sin(Fp(1))*Fy(3))*Fz(5))/(Fz(3) + g)^2))/(((cos(Fp(1))*Fx(3) + sin(Fp(1))*Fy(3))^2/(Fz(3) + g)^2 + 1)*((cos(Fp(1))*Fy(3) - sin(Fp(1))*Fx(3))^2/((Fz(3) + g)^2 + (cos(Fp(1))*Fx(3) + sin(Fp(1))*Fy(3))^2) + 1)^(1/2)*((Fz(3) + g)^2 + (cos(Fp(1))*Fx(3) + sin(Fp(1))*Fy(3))^2)^(1/2)) - (((sin(Fp(1))*Fy(4) + cos(Fp(1))*Fx(4) + cos(Fp(1))*Fy(3)*Fp(2) - sin(Fp(1))*Fx(3)*Fp(2))/(Fz(3) + g) - ((cos(Fp(1))*Fx(3) + sin(Fp(1))*Fy(3))*Fz(4))/(Fz(3) + g)^2)*(sin(Fp(1))*Fx(4) - cos(Fp(1))*Fy(4) + cos(Fp(1))*Fx(3)*Fp(2) + sin(Fp(1))*Fy(3)*Fp(2)))/(((cos(Fp(1))*Fx(3) + sin(Fp(1))*Fy(3))^2/(Fz(3) + g)^2 + 1)*((cos(Fp(1))*Fy(3) - sin(Fp(1))*Fx(3))^2/((Fz(3) + g)^2 + (cos(Fp(1))*Fx(3) + sin(Fp(1))*Fy(3))^2) + 1)^(1/2)*((Fz(3) + g)^2 + (cos(Fp(1))*Fx(3) + sin(Fp(1))*Fy(3))^2)^(1/2)) + (((sin(Fp(1))*Fy(4) + cos(Fp(1))*Fx(4) + cos(Fp(1))*Fy(3)*Fp(2) - sin(Fp(1))*Fx(3)*Fp(2))/(Fz(3) + g) - ((cos(Fp(1))*Fx(3) + sin(Fp(1))*Fy(3))*Fz(4))/(Fz(3) + g)^2)*(cos(Fp(1))*Fy(3) - sin(Fp(1))*Fx(3))*(((2*(Fz(3) + g)*Fz(4) + 2*(cos(Fp(1))*Fx(3) + sin(Fp(1))*Fy(3))*(sin(Fp(1))*Fy(4) + cos(Fp(1))*Fx(4) + cos(Fp(1))*Fy(3)*Fp(2) - sin(Fp(1))*Fx(3)*Fp(2)))*(cos(Fp(1))*Fy(3) - sin(Fp(1))*Fx(3))^2)/((Fz(3) + g)^2 + (cos(Fp(1))*Fx(3) + sin(Fp(1))*Fy(3))^2)^2 + (2*(cos(Fp(1))*Fy(3) - sin(Fp(1))*Fx(3))*(sin(Fp(1))*Fx(4) - cos(Fp(1))*Fy(4) + cos(Fp(1))*Fx(3)*Fp(2) + sin(Fp(1))*Fy(3)*Fp(2)))/((Fz(3) + g)^2 + (cos(Fp(1))*Fx(3) + sin(Fp(1))*Fy(3))^2)))/(2*((cos(Fp(1))*Fx(3) + sin(Fp(1))*Fy(3))^2/(Fz(3) + g)^2 + 1)*((cos(Fp(1))*Fy(3) - sin(Fp(1))*Fx(3))^2/((Fz(3) + g)^2 + (cos(Fp(1))*Fx(3) + sin(Fp(1))*Fy(3))^2) + 1)^(3/2)*((Fz(3) + g)^2 + (cos(Fp(1))*Fx(3) + sin(Fp(1))*Fy(3))^2)^(1/2)) - (((2*(cos(Fp(1))*Fx(3) + sin(Fp(1))*Fy(3))*(sin(Fp(1))*Fy(4) + cos(Fp(1))*Fx(4) + cos(Fp(1))*Fy(3)*Fp(2) - sin(Fp(1))*Fx(3)*Fp(2)))/(Fz(3) + g)^2 - (2*(cos(Fp(1))*Fx(3) + sin(Fp(1))*Fy(3))^2*Fz(4))/(Fz(3) + g)^3)*((sin(Fp(1))*Fy(4) + cos(Fp(1))*Fx(4) + cos(Fp(1))*Fy(3)*Fp(2) - sin(Fp(1))*Fx(3)*Fp(2))/(Fz(3) + g) - ((cos(Fp(1))*Fx(3) + sin(Fp(1))*Fy(3))*Fz(4))/(Fz(3) + g)^2)*(cos(Fp(1))*Fy(3) - sin(Fp(1))*Fx(3)))/(((cos(Fp(1))*Fx(3) + sin(Fp(1))*Fy(3))^2/(Fz(3) + g)^2 + 1)^2*((cos(Fp(1))*Fy(3) - sin(Fp(1))*Fx(3))^2/((Fz(3) + g)^2 + (cos(Fp(1))*Fx(3) + sin(Fp(1))*Fy(3))^2) + 1)^(1/2)*((Fz(3) + g)^2 + (cos(Fp(1))*Fx(3) + sin(Fp(1))*Fy(3))^2)^(1/2)) - ((2*(Fz(3) + g)*Fz(4) + 2*(cos(Fp(1))*Fx(3) + sin(Fp(1))*Fy(3))*(sin(Fp(1))*Fy(4) + cos(Fp(1))*Fx(4) + cos(Fp(1))*Fy(3)*Fp(2) - sin(Fp(1))*Fx(3)*Fp(2)))*((sin(Fp(1))*Fy(4) + cos(Fp(1))*Fx(4) + cos(Fp(1))*Fy(3)*Fp(2) - sin(Fp(1))*Fx(3)*Fp(2))/(Fz(3) + g) - ((cos(Fp(1))*Fx(3) + sin(Fp(1))*Fy(3))*Fz(4))/(Fz(3) + g)^2)*(cos(Fp(1))*Fy(3) - sin(Fp(1))*Fx(3)))/(2*((cos(Fp(1))*Fx(3) + sin(Fp(1))*Fy(3))^2/(Fz(3) + g)^2 + 1)*((cos(Fp(1))*Fy(3) - sin(Fp(1))*Fx(3))^2/((Fz(3) + g)^2 + (cos(Fp(1))*Fx(3) + sin(Fp(1))*Fy(3))^2) + 1)^(1/2)*((Fz(3) + g)^2 + (cos(Fp(1))*Fx(3) + sin(Fp(1))*Fy(3))^2)^(3/2));

	d_omega = [dwx; dwy; dwz];

    TauX = Jx*dwx + (Jz - Jy)*wy*wz;
    TauY = Jy*dwy + (Jx - Jz)*wx*wz;
    TauZ = Jz*dwz + (Jy - Jx)*wx*wy;

	Tau = [TauX; TauY; TauZ];

== matlab function project/Drone Model/Drone Model ==
  settings: updateMethod=DISCRETE
  data: T input; Tau input; RPY input; acc output; dw output; omega input; m data_store_memory; Jz data_store_memory; Jy data_store_memory; Jx data_store_memory; g data_store_memory
function [acc, dw] = drone(T, Tau, RPY, omega)
    global m;
    global g;
    global Jz;
    global Jy;
    global Jx;

	Fi = RPY(1);
	Theta = RPY(2);
	Psi = RPY(3);

	TauX = Tau(1);
	TauY = Tau(2);
	TauZ = Tau(3);

	wx = omega(1);
	wy = omega(2);
	wz = omega(3);

	x_dd = T / m * ( cos(Psi)*sin(Theta)*cos(Fi) + sin(Psi)*sin(Fi) );
	y_dd = T / m * ( sin(Psi)*sin(Theta)*cos(Fi) - cos(Psi)*sin(Fi) );
	z_dd = T / m * ( cos(Theta)*cos(Fi) ) - g;
	acc = [x_dd; y_dd; z_dd];

    dwx = ( TauX - (Jz - Jy)*wy*wz ) / Jx;
    dwy = ( TauY - (Jx - Jz)*wx*wz ) / Jy;
    dwz = ( TauZ - (Jy - Jx)*wx*wy ) / Jz;
	dw = [ dwx; dwy; dwz ];
end

== matlab function project/MATLAB Function ==
  data: pos input; W data_store_memory
function plot_position(pos)
	global W;
	persistent X;
	persistent Y;
	persistent Z;

	if isempty(X)
		X = [];
		Y = [];
		Z = [];
	end
	
	X = [X pos(1)];
	Y = [Y pos(2)];
	Z = [Z pos(3)];
	
	figure(2)
	plot3(W(:, 1), W(:, 2), W(:, 3), 'o', Color="blue", MarkerSize=5, MarkerFaceColor="blue")
	hold on

	plot3(X, Y, Z, "LineWidth", 2);
	grid on
	hold off

== matlab function project/Drone Model/Outer Loop Control ==
  data: v input; p input; p_ref input; v_ref input; R_des output; a_ref input; R input; c_des output; omega_des output; d_omega_des output; omega_ref input; d_omega_ref input
function [R_des, c_des, omega_des, d_omega_des] = outer(v, p, p_ref, v_ref, a_ref, R, omega_ref, d_omega_ref)
	g = 9.81;
	K_pos = 0.1; % diag([1 1 1])
	K_vel = 0.01; % diag([1 1 1])
	epsilon = 0.00001;
	e_z = [0; 0; 1];
	p_ref_z = p_ref(3);
	y_c = [-sin(p_ref_z); cos(p_ref_z); 0]
	z_B = R(:, 3)
	p_rp = 0.2;
	p_y = 1;

	pd = -p + p_ref;
	vd = -v + v_ref;

	a_fb = -K_pos * pd - K_vel * vd;
	a_des = a_fb + a_ref + g*e_z;

	zB_des = a_des / norm(a_des + epsilon)
	
	xB_des = cross(y_c, zB_des) / norm(cross(y_c, zB_des))
	yB_des = cross(zB_des, xB_des) 

	c_des = a_des' * z_B

	alpha = acos(dot(z_B, xB_des))
	
	n_nominator = cross(z_B, zB_des)
	n_denominator = norm(cross(z_B, zB_des)) + 0.00001
	n = cross(z_B, zB_des) / n_denominator
	n_B = R \ n
    q_e_rp = [1 0 0 0];

	if alpha ~= 0
    	q_e_rp = [cos(alpha/2); n_B * sin(alpha/2)]';
	end
	
	omega_x_fb = 2 * p_rp * q_e_rp(2)
	omega_y_fb = 2 * p_rp * q_e_rp(3)
	if q_e_rp(1) < 0
    	omega_x_fb = -1*omega_x_fb
    	omega_y_fb = -1*omega_y_fb
	end

	% Yaw

	if zB_des < 0
    	xB_des = -xB_des;
	end
	
	R_des = [xB_des, yB_des, zB_des];
	
	q = rotm2quat(R);
	q_des = rotm2quat(R_des);
	
	q_e_y = quatmultiply(quatconj(quatmultiply(q, q_e_rp)), q_des);
	
	if q_e_y(1) >= 0
    	omega_z_fb = 2 *  p_y * q_e_y(4);
	else
    	omega_z_fb = -2 * p_y * q_e_y(4);
	end
	
	omega_fb = [omega_x_fb; omega_y_fb; omega_z_fb]
	
	
	omega_des = omega_fb + omega_ref
	
	% fifth step
	d_omega_des = d_omega_ref;
